simulink model "state_space"  (R2021a)
settings: Solver=VariableStepAuto  StartTime=0.0  StopTime=10.0  RelTol=1e-3
undefined symbols (not defined in the file): a, B, C, D, K
settings Model: Creator=shiva  LastModifiedBy=shiva

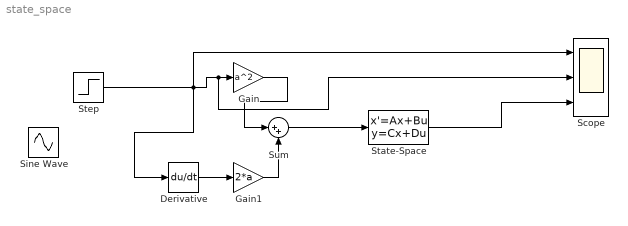
== system state_space ==
  Derivative : Derivative
  Gain : Gain  Gain=a^2
  Gain1 : Gain  Gain=2*a
  Scope : Scope  NumInputPorts=3
  Sine Wave : Sin  SampleTime=0
  State-Space : StateSpace  A=K  B=B  C=C  D=D  InitialCondition=[0 0 0 0 0 0]  ParameterTunability=Unconstrained
  Step : Step  SampleTime=0
  Sum : Sum  Inputs=|++
  wires:
  Sum/1 -> State-Space/1
  State-Space/1 -> Scope/3
  Derivative/1 -> Gain1/1
  Gain1/1 -> Sum/2
  Step/1 -> Derivative/1, Scope/2, Gain/1, Scope/1
  Gain/1 -> Sum/1
